simulink model "Nominal"  (R2019b)
settings: Solver=VariableStepAuto  StartTime=0.0  StopTime=10.0  RelTol=1e-3
undefined symbols (not defined in the file): Ki, Kp, Kt_r, l, m
settings Model: Creator=ZYT  LastModifiedBy=ZYT

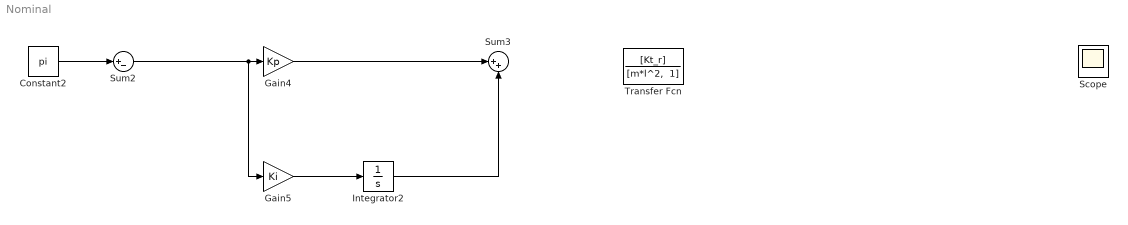
== system Nominal ==
  Constant2 : Constant  Value=pi
  Gain4 : Gain  Gain=Kp
  Gain5 : Gain  Gain=Ki
  Integrator2 : Integrator
  Scope : Scope
  Sum2 : Sum  Inputs=|+-
  Sum3 : Sum  Inputs=|++
  Transfer Fcn : TransferFcn  Numerator=[Kt_r]  Denominator="[m*l^2,  1]"
  wires:
  Sum2/1 -> Gain5/1, Gain4/1
  Constant2/1 -> Sum2/1
  Gain4/1 -> Sum3/1
  Gain5/1 -> Integrator2/1
  Integrator2/1 -> Sum3/2
